simulink model "ControlMotores"  (R2023b)
settings: Solver=VariableStepAuto  StartTime=0.0  StopTime=10.0  RelTol=1e-3
libraries: arduinolib x6, simulink x2
settings Model: Creator=manu_  LastModifiedBy=manu_

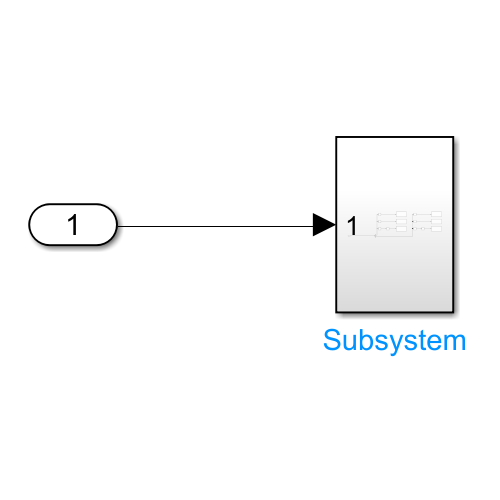
[thumbnail: Simulink's stored preview of the top-level diagram]
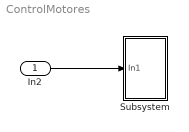
== system ControlMotores ==
  In2 : Inport
  Subsystem : Subsystem
  wires:
  In2/1 -> Subsystem/1(In1)

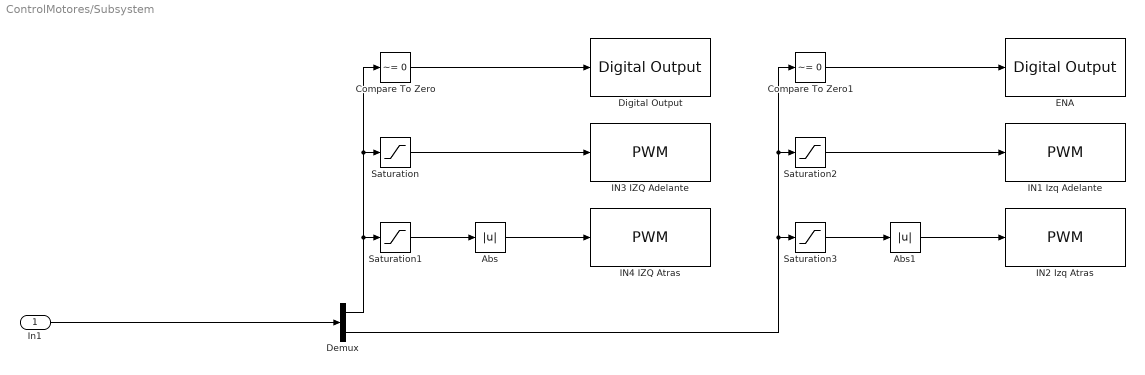
== system ControlMotores/Subsystem ==
  In1 : Inport
  Abs : Abs  SaturateOnIntegerOverflow=off
  Abs1 : Abs  SaturateOnIntegerOverflow=off
  Compare To Zero : simulink/Logic and Bit Operations/Compare To Zero  relop=~=  OutDataTypeStr=boolean
  Compare To Zero1 : simulink/Logic and Bit Operations/Compare To Zero  relop=~=  OutDataTypeStr=boolean
  Demux : Demux  Outputs=2
  Digital Output : arduinolib/Digital Output  pinNumber=13  Direction=output  blockPlatform=arduino
  ENA : arduinolib/Digital Output  pinNumber=8  Direction=output  blockPlatform=arduino
  IN1 Izq Adelante : arduinolib/PWM  pinNumber=9  frequencyType=Default  desiredFrequency=490.2  achievableFrequency=490.2
  IN2 Izq Atras : arduinolib/PWM  pinNumber=10  frequencyType=Default  desiredFrequency=490.2  achievableFrequency=490.2
  IN3 IZQ Adelante : arduinolib/PWM  pinNumber=11  frequencyType=Default  desiredFrequency=490.2  achievableFrequency=490.2
  IN4 IZQ Atras : arduinolib/PWM  pinNumber=12  frequencyType=Default  desiredFrequency=490.2  achievableFrequency=490.2
  Saturation : Saturate  UpperLimit=255  LowerLimit=0
  Saturation1 : Saturate  UpperLimit=0  LowerLimit=-255
  Saturation2 : Saturate  UpperLimit=255  LowerLimit=0
  Saturation3 : Saturate  UpperLimit=0  LowerLimit=-255
  wires:
  Demux/2 -> Compare To Zero1/1, Saturation2/1, Saturation3/1
  Demux/1 -> Compare To Zero/1, Saturation/1, Saturation1/1
  Saturation3/1 -> Abs1/1
  Compare To Zero/1 -> Digital Output/1
  Compare To Zero1/1 -> ENA/1
  Abs1/1 -> IN2 Izq Atras/1
  In1/1 -> Demux/1
  Abs/1 -> IN4 IZQ Atras/1
  Saturation1/1 -> Abs/1
  Saturation/1 -> IN3 IZQ Adelante/1
  Saturation2/1 -> IN1 Izq Adelante/1
